simulink model "kalman_filter"  (R2022b)
settings: Solver=VariableStepAuto  StartTime=0.0  StopTime=10.0  RelTol=1e-3
undefined symbols (not defined in the file): Discrete, Time
libraries: ctrlSharedLib x1
settings Model: Creator=miakho  LastModifiedBy=miakho

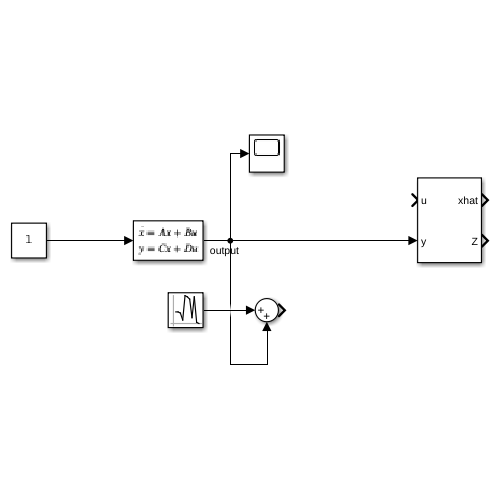
[thumbnail: Simulink's stored preview of the top-level diagram]
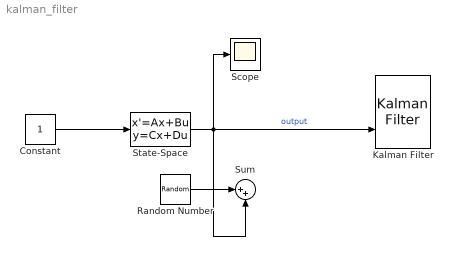
== system kalman_filter ==
  Constant : Constant
  Kalman Filter : ctrlSharedLib/Kalman Filter  TimeDomain=Discrete-Time  UseCurrentEstimator=on  ModelSource=LTI State-Space Variable  ModelSourceVariable=ss(0.95,1,1,0,1)  A=0.95  B=1  C=1  D=0  NumberOfStates=1  NumberOfInputs=1  NumberOfOutputs=1  InitialEstimateSource=Dialog  X0=0  P0=10  UseK=off  UseGH=off  NumberOfProcessNoiseInputs=1  G=1  TimeInvariantG=on  H=0  TimeInvariantH=on  Q=0.05  TimeInvariantQ=on  R=1  TimeInvariantR=on  N=0  TimeInvariantN=on  AddInputPort=on  AddEnablePort=off  OutputEstimatedY=off  OutputP=on  Ts=-1
  Random Number : RandomNumber  SampleTime=0.1
  Scope : Scope
  State-Space : StateSpace  InitialCondition=0  ContinuousStateAttributes={'position'}
  Sum : Sum  Inputs=|++
  wires:
  Constant/1 -> State-Space/1
  State-Space/1 -> Scope/1, Kalman Filter/2, Sum/2  "output"
  Random Number/1 -> Sum/1
